simulink model "MMKF_example_sim"  (R2019b)
settings: Solver=FixedStepAuto  StartTime=0.0  StopTime=nT*Ts  FixedStep=Ts  RelTol=1e-3
values from neighbouring files (symbols this model uses):
  A = Model.A    [GPB1_estimation.m]    (also in GPB2_estimation.m; MKFObserverRODD.m = repmat({A}, 1, nj); MKFObserverSF.m = repmat({A}, 1, nj); MKFObserverSF95.m = repmat({A}, 1, nj))
  Bu = repmat({Bu}, 1, nj)    [MKFObserverRODD.m]    (also in MKFObserverSF.m; MKFObserverSF95.m; MKFObserverSF98.m; MKFObserverSF_RODD.m = model.B(:, u_meas))
  C = Model.C    [GPB1_estimation.m]    (also in GPB2_estimation.m; MKFObserverDI.m = obj.filters{f}.C; MKFObserverF.m = obj.filters{f}.C; MKFObserverGPB1.m = obj.filters{f}.C)
  Du = repmat({Du}, 1, nj)    [MKFObserverRODD.m]    (also in MKFObserverSF.m; MKFObserverSF95.m; MKFObserverSF_RODD.m = model.D(:, u_meas))
  N = size(Model.A,1)    [GPB1_estimation.m]    (also in GPB2_estimation.m = size(Model.A{1}, 1))
  x0 = zeros(n, 1)    [AbstractLinearFilter.m]    (also in EKF_filter.m; EKF_observer.m; KalmanFilter.m; KalmanFilterJS.m = zeros(obj.n, 1))
undefined symbols (not defined in the file or in its folder): Discrete, KF1, Time, Ts
libraries: ctrlSharedLib x1
settings Model: Creator=Andre  LastModifiedBy=billtubbs
settings DataIOCC: ReturnWorkspaceOutputs=off
settings DebuggingCC: ArithmeticOperatorsInVariantConditions=warning
settings SFSimCC: SimUseLocalCustomCode=off  CustomCodeUndefinedFunction=UseInterfaceOnly
settings RTWCC: RTWUseLocalCustomCode=off

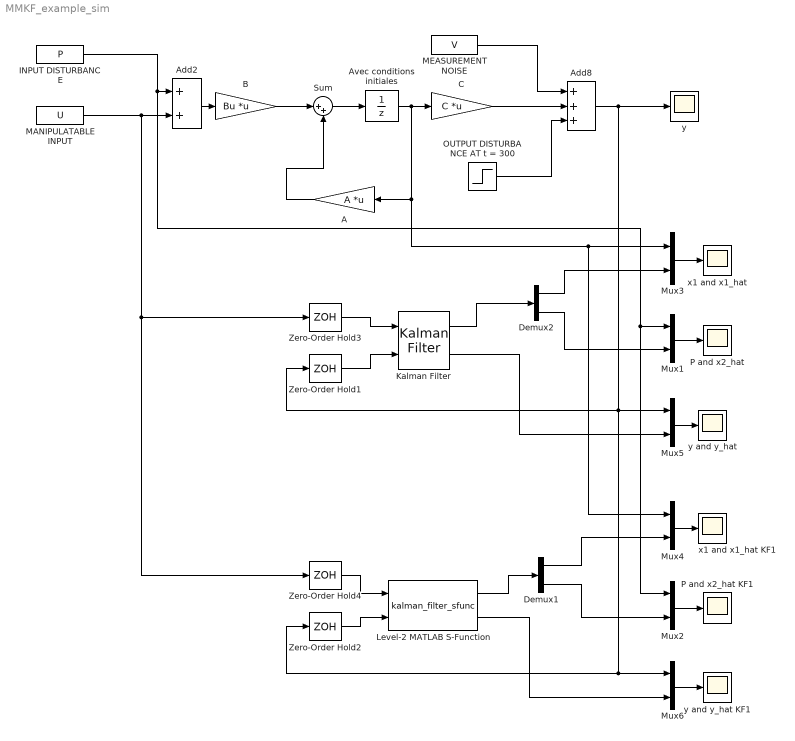
== system MMKF_example_sim ==
  A : Gain  Gain=A  Multiplication=Matrix(K*u)
  Add2 : Sum
  Add8 : Sum  Inputs=+++
  Avec conditions initiales : UnitDelay  InitialCondition=x0  SampleTime=Ts  HasFrameUpgradeWarning=on
  B : Gain  Gain=Bu  Multiplication=Matrix(K*u)
  C : Gain  Gain=C  Multiplication=Matrix(K*u)
  Demux1 : Demux  Outputs=2
  Demux2 : Demux  Outputs=2
  INPUT DISTURBANCE : FromWorkspace  VariableName=P  SampleTime=Ts
  Kalman Filter : ctrlSharedLib/Kalman Filter  TimeDomain=Discrete-Time  UseCurrentEstimator=off  ModelSource=Individual A, B, C, D matrices  ModelSourceVariable=G  A=A  B=Bu  C=C  D=Du  NumberOfStates=1  NumberOfInputs=1  NumberOfOutputs=1  InitialEstimateSource=Dialog  X0=[0; 0]  P0=10  UseK=off  UseGH=off  NumberOfProcessNoiseInputs=1  G=Gkf  TimeInvariantG=on  H=Hkf  TimeInvariantH=on  Q=KF1.Q  TimeInvariantQ=on  R=KF1.R  TimeInvariantR=on  N=N  TimeInvariantN=on  AddInputPort=on  AddEnablePort=off  OutputEstimatedY=on  OutputP=off  Ts=KF1.Ts
      settings: SourceProductBaseCode=CT
  Level-2 MATLAB S-Function : M-S-Function  FunctionName=kalman_filter_sfunc  Parameters=KF1
  MANIPULATABLE INPUT : FromWorkspace  VariableName=U  SampleTime=Ts
  MEASUREMENT NOISE : FromWorkspace  VariableName=V  SampleTime=Ts
  Mux{1..6} (6 alike) : Mux  Inputs=2
  OUTPUT DISTURBANCE AT t = 300 : Step  Time=300  After=0  SampleTime=0
  P and x2_hat : Scope
  P and x2_hat KF1 : Scope
  Sum : Sum  Inputs=|++
  Zero-Order Hold{1..4} (4 alike) : ZeroOrderHold  SampleTime=Ts
  x1 and x1_hat : Scope
  x1 and x1_hat KF1 : Scope
  y : Scope
  y and y_hat : Scope
  y and y_hat KF1 : Scope
  wires:
  A/1 -> Sum/2
  Mux3/1 -> x1 and x1_hat/1
  Mux1/1 -> P and x2_hat/1
  Sum/1 -> Avec conditions initiales/1
  B/1 -> Sum/1
  OUTPUT DISTURBANCE AT t = 300/1 -> Add8/3
  Avec conditions initiales/1 -> C/1, Mux4/1, Mux3/1, A/1
  C/1 -> Add8/2
  MEASUREMENT NOISE/1 -> Add8/1
  Kalman Filter/2 -> Mux5/2
  Mux5/1 -> y and y_hat/1
  Kalman Filter/1 -> Demux2/1
  Demux2/1 -> Mux3/2
  Demux2/2 -> Mux1/2
  Add8/1 -> Zero-Order Hold2/1, Mux6/1, Zero-Order Hold1/1, Mux5/1, y/1
  MANIPULATABLE INPUT/1 -> Add2/2, Zero-Order Hold4/1, Zero-Order Hold3/1
  Zero-Order Hold3/1 -> Kalman Filter/1
  Zero-Order Hold1/1 -> Kalman Filter/2
  INPUT DISTURBANCE/1 -> Mux2/1, Mux1/1, Add2/1
  Add2/1 -> B/1
  Zero-Order Hold4/1 -> Level-2 MATLAB S-Function/1
  Zero-Order Hold2/1 -> Level-2 MATLAB S-Function/2
  Mux6/1 -> y and y_hat KF1/1
  Level-2 MATLAB S-Function/2 -> Mux6/2
  Mux4/1 -> x1 and x1_hat KF1/1
  Mux2/1 -> P and x2_hat KF1/1
  Level-2 MATLAB S-Function/1 -> Demux1/1
  Demux1/1 -> Mux4/2
  Demux1/2 -> Mux2/2
